simulink model "ms2"  (R2023b)
settings: Solver=FixedStepDiscrete  StartTime=0.0  StopTime=10.0  FixedStep=1e-3  RelTol=1e-3  EnableMultiTasking=on
settings Model: DataDictionary=common.sldd  Creator=mfussi  LastModifiedBy=mfussi
settings SolverCC: AutoInsertRateTranBlk=on  InsertRTBMode=Never (minimum delay)
settings DataIOCC: SaveOutput=off  SignalLogging=off  DSMLogging=off  StreamToWks=off  SaveTime=off  ReturnWorkspaceOutputs=off
settings OptimizationCC: DefaultParameterBehavior=Inlined  UseDivisionForNetSlopeComputation=on  GainParamInheritBuiltInType=on  UseFloatMulNetSlope=on  InlineInvariantSignals=on  EnhancedBackFolding=on  NoFixptDivByZeroProtection=on  EfficientFloat2IntCast=on  OptimizeBlockOrder=speed  DifferentSizesBufferReuse=on  OptimizationCustomize=off  EfficientTunableParamExpr=on
settings DebuggingCC: ParameterTunabilityLossMsg=error
settings HardwareCC: ProdBitPerPointer=32  ProdBitPerSizeT=32  ProdBitPerPtrDiffT=32  ProdLargestAtomicInteger=Long  ProdLargestAtomicFloat=Double  ProdWordSize=32  ProdLongLongMode=on  ProdHWDeviceType=ARM Compatible->ARM Cortex-M
settings SFSimCC: MATLABDynamicMemAlloc=off
settings SFSimCC: SimCustomHeaderCode=|
  | #include "rtw_enable_disable_motors.h"
  | #include "rtw_motor_config.h"
settings SFSimCC: SimUserSources=|
  | rtw_enable_disable_motors.c
  | rtw_motor_config.c
settings RTWCC: Description=Embedded Coder  SystemTargetFile=ert.tlc  GenCodeOnly=on  TemplateMakefile=ert_default_tmf  RTWUseSimCustomCode=on
settings RTWCC: CustomHeaderCode=|
  | #include "rtw_enable_disable_motors.h"
  | #include "rtw_motor_config.h"
settings RTWCC: CustomSource=|
  | rtw_enable_disable_motors.c
  | rtw_motor_config.c
settings CodeAppCC: ForceParamTrailComments=on  IgnoreCustomStorageClasses=off  OperatorAnnotations=on  SimulinkDataObjDesc=on  SFDataObjDesc=on  InsertBlockDesc=on
settings ERTTargetCC: TargetLangStandard=C99 (ISO)  CodeReplacementLibrary=ARM Cortex-M,iCubTech  GenerateSampleERTMain=on  SuppressErrorStatus=on  CodeInterfacePackaging=Reusable function  SupportNonFinite=off  InlinedParameterPlacement=NonHierarchical  RootIOFormat=Structure reference  ERTCustomFileTemplate=example_file_process.tlc

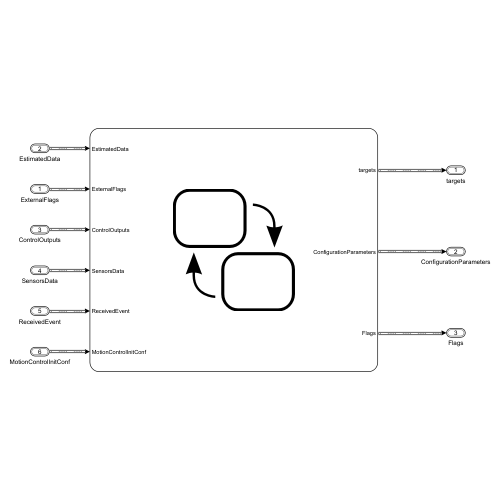
[thumbnail: Simulink's stored preview of the top-level diagram]
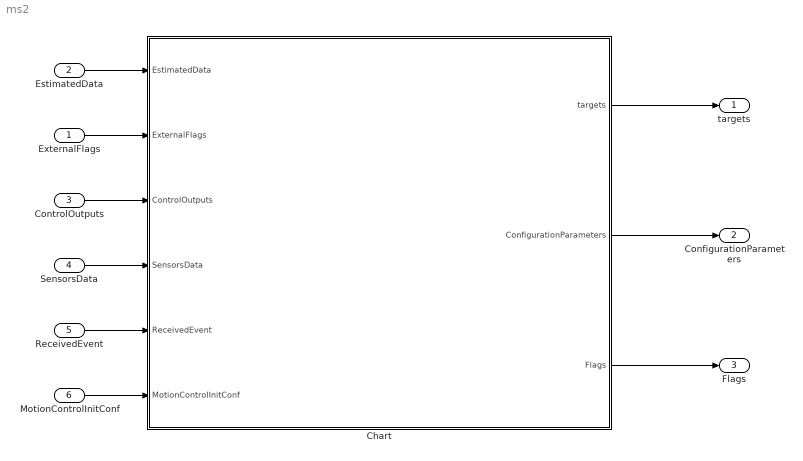
== system ms2 ==
  ExternalFlags : Inport  OutDataTypeStr=Bus: ExternalFlags  BusOutputAsStruct=on
  EstimatedData : Inport  Port=2  OutDataTypeStr=Bus: EstimatedData  BusOutputAsStruct=on
  ControlOutputs : Inport  Port=3  OutDataTypeStr=Bus: FOCOutputs  BusOutputAsStruct=on
  SensorsData : Inport  Port=4  OutDataTypeStr=Bus: SensorsData  BusOutputAsStruct=on
  ReceivedEvent : Inport  Port=5  OutDataTypeStr=Bus: SupervisorReceivedEvents  BusOutputAsStruct=on
  MotionControlInitConf : Inport  Port=6  OutDataTypeStr=Bus: ActuatorConfiguration  BusOutputAsStruct=on
  Chart : Stateflow chart  TreatAsAtomicUnit=on
  targets : Outport  OutDataTypeStr=Bus: Targets  BusOutputAsStruct=on
  ConfigurationParameters : Outport  Port=2  OutDataTypeStr=Bus: ActuatorConfiguration  BusOutputAsStruct=on
  Flags : Outport  Port=3  OutDataTypeStr=Bus: Flags  BusOutputAsStruct=on
  wires:
  ExternalFlags/1 -> Chart/2(ExternalFlags)
  EstimatedData/1 -> Chart/1(EstimatedData)
  ControlOutputs/1 -> Chart/3(ControlOutputs)
  SensorsData/1 -> Chart/4(SensorsData)
  ReceivedEvent/1 -> Chart/5(ReceivedEvent)
  Chart/1(targets) -> targets/1
  Chart/2(ConfigurationParameters) -> ConfigurationParameters/1
  Chart/3(Flags) -> Flags/1
  MotionControlInitConf/1 -> Chart/6(MotionControlInitConf)

== stateflow chart ms2/Chart ==
  settings: updateMethod=DISCRETE  sampleTime=1e-3
  state FaultsManager [parallel]
    settings: executionOrder=1
    state FaultButton [parallel]
      settings: executionOrder=2
      state NoFault
        entry:
        isFaultButtonPressed = false;
      state ButtonPressed
        entry:
        isFaultButtonPressed = true;
        send(faultButtonPressed, ControlModeHandler);
      (default) -> FaultsManager.FaultButton.NoFault
      ButtonPressed -> FaultsManager.FaultButton.NoFault : [hasChangedTo(ExternalFlags.fault_button, false)]
      FaultsManager.FaultButton.NoFault -> ButtonPressed : [hasChangedTo(ExternalFlags.fault_button, true)]
    state HWFaults [parallel]
      settings: executionOrder=1
      state NoFault
        entry:
        //MotorFaultFlags.overCurrent=0;
      state LimitNonConfigured
      state OverCurrentFault
        entry:
        //MotorFaultFlags.overCurrent=1;
        isInFault=true;
        send(hwFault, ControlModeHandler);
      (default) -> LimitNonConfigured
      LimitNonConfigured -> FaultsManager.HWFaults.NoFault : [areLimitsSet==true]
      FaultsManager.HWFaults.NoFault -> OverCurrentFault : [abs(EstimatedData.Iq_filtered) >= ConfigurationParameters.thresholds.motorOverloadCurrents]
      OverCurrentFault -> FaultsManager.HWFaults.NoFault : [abs(EstimatedData.Iq_filtered) < ConfigurationParameters.thresholds.motorOverloadCurrents]
  state ControlModeHandler [parallel]
    settings: executionOrder=3
    state NotConfigured
      entry:
      Flags.control_mode = ControlModes.NotConfigured;
      // rtw_disableMotor();
    state Idle
      entry:
      Flags.control_mode = ControlModes.Idle;
      // rtw_disableMotor();
      //rtw_enableMotor()
      //this updates the targets value
      send(ControlModeSetpointChange, TargetsManager);
    state Position
      entry:
      Flags.control_mode = ControlModes.Position;
      newSetpoint=SensorsData.jointpositions;
      send(ControlModeSetpointChange, TargetsManager);
    state Current
      entry:
      Flags.control_mode = ControlModes.Current;
      send(ControlModeSetpointChange, TargetsManager);
    state HWFault
      entry:
      Flags.control_mode = ControlModes.HwFaultCM;
      // rtw_disableMotor();
      //this updates the targets value
      send(ControlModeSetpointChange, TargetsManager);
    state Voltage
      entry:
      Flags.control_mode = ControlModes.Voltage;
      send(ControlModeSetpointChange, TargetsManager);
    note: IMPORTANT:
        | Currently we use IDLE command to exit from HWFault state,
        | but We should use FORCE_IDLE command when it will be implemented
    state Velocity
      entry:
      Flags.control_mode = ControlModes.Velocity;
      newSetpoint=0;
      send(ControlModeSetpointChange, TargetsManager);
    (junction 223) -> (junction 199)
    (junction 226) -> (junction 223) [order 1] : initialControlModeTrigger
    (junction 199) -> (junction 233)
    (default) -> (junction 226)
    (junction 226) -> NotConfigured [order 2]
    NotConfigured -> (junction 229) [order 1] : initialControlModeTrigger
        | {requiredControlMode = ControlModes.Idle;}
    (junction 229) -> (junction 233)
    (junction 227) -> (junction 233)
    (junction 282) -> (junction 227)
    (junction 273) -> (junction 229)
    (junction 233) -> Idle
    HWFault -> NotConfigured [order 1] : [!isInFault && isReqMode(ControlModes.Idle) && !isConfigurationSet()]
    NotConfigured -> HWFault [order 2] : [isInFault]
    (junction 228) -> Idle
    (junction 236) -> (junction 228)
    Idle -> (junction 230) [order 2]
    (junction 230) -> (junction 237)
    (junction 234) -> Idle : SetCtrlMode[isReqMode(ControlModes.Idle)]
    (junction 235) -> (junction 234) [order 2]
    (junction 224) -> Idle : SetCtrlMode[isReqMode(ControlModes.Idle)]
    (junction 243) -> (junction 224) [order 2]
    (junction 231) -> Idle : SetCtrlMode[isReqMode(ControlModes.Idle)]
    (junction 241) -> (junction 231) [order 2]
    Idle -> (junction 232) [order 1] : [isInFault || isFaultButtonPressed]
    (junction 232) -> (junction 225)
    (junction 225) -> (junction 248)
    Position -> (junction 236) [order 3] : SetCtrlMode[isReqMode(ControlModes.Idle)]
    (junction 237) -> Position [order 1] : SetCtrlMode[isReqMode(ControlModes.Position)]
    (junction 237) -> (junction 244) [order 2]
    (junction 235) -> Position [order 1] : SetCtrlMode[isReqMode(ControlModes.Position)]
    (junction 245) -> (junction 235)
    Position -> (junction 242) [order 2] : SetCtrlMode[!isReqMode(ControlModes.Idle)]
    (junction 242) -> (junction 240)
    (junction 243) -> Position [order 1] : SetCtrlMode[isReqMode(ControlModes.Position)]
    (junction 247) -> (junction 243) [order 2]
    (junction 241) -> Position [order 1] : SetCtrlMode[isReqMode(ControlModes.Position)]
    (junction 255) -> (junction 241) [order 2]
    Position -> (junction 238) [order 1] : [isInFault || isFaultButtonPressed]
    (junction 238) -> (junction 248)
    (junction 248) -> (junction 259)
    (junction 244) -> Current [order 1] : SetCtrlMode[isReqMode(ControlModes.Current)]{ newSetpoint=0; }
    (junction 244) -> (junction 278) [order 2]
    Current -> (junction 245) [order 3]
    (junction 240) -> (junction 239) [order 1] : SetCtrlMode[isReqMode(ControlModes.Current)]
    (junction 239) -> Current : {newSetpoint=ControlOutputs.Iq_fbk;}
    (junction 240) -> (junction 258) [order 2]
    (junction 247) -> (junction 246) [order 1] : SetCtrlMode[isReqMode(ControlModes.Current)]
    (junction 246) -> (junction 276)
    (junction 263) -> (junction 247)
    Current -> (junction 275) [order 2] : SetCtrlMode[!isReqMode(ControlModes.Idle) && !isReqMode(ControlModes.Position)]
    (junction 275) -> (junction 257)
    (junction 276) -> Current : {newSetpoint=ControlOutputs.Iq_fbk;}
    (junction 255) -> (junction 276) [order 1] : SetCtrlMode[isReqMode(ControlModes.Current)]
    HWFault -> (junction 273) [order 2] : SetCtrlMode[!isInFault && isReqMode(ControlModes.Idle)]
    (junction 261) -> (junction 255) [order 2]
    Current -> (junction 267) [order 1] : [isInFault || isFaultButtonPressed]
    (junction 267) -> (junction 259)
    (junction 259) -> (junction 279)
    (junction 268) -> HWFault
    (junction 278) -> Voltage [order 1] : SetCtrlMode[isReqMode(ControlModes.Voltage)]{newSetpoint=0; }
    (junction 278) -> (junction 251) [order 2]
    (junction 258) -> (junction 277) [order 1] : SetCtrlMode[isReqMode(ControlModes.Voltage)]
    (junction 277) -> Voltage : {newSetpoint=ControlOutputs.Vq;}
    (junction 258) -> (junction 251) [order 2]
    (junction 283) -> (junction 277)
    Voltage -> (junction 263) [order 2]
    (junction 257) -> (junction 283) [order 1] : SetCtrlMode[isReqMode(ControlModes.Voltage)]
    (junction 257) -> (junction 251) [order 2]
    Voltage -> (junction 251) [order 3]
    (junction 269) -> Voltage : {newSetpoint=ControlOutputs.Vq;}
    (junction 261) -> (junction 269) [order 1] : SetCtrlMode[isReqMode(ControlModes.Voltage)]
    (junction 265) -> (junction 261) : SetCtrlMode[!isReqMode(ControlModes.Velocity)]
    Voltage -> (junction 260) [order 1] : [isInFault || isFaultButtonPressed]
    (junction 260) -> (junction 279)
    (junction 279) -> (junction 253)
    (junction 251) -> Velocity : SetCtrlMode[isReqMode(ControlModes.Velocity)]
    Velocity -> (junction 265) [order 2]
    Velocity -> (junction 280) [order 1] : [isInFault || isFaultButtonPressed]
    (junction 280) -> (junction 253)
    (junction 253) -> (junction 281)
    (junction 281) -> (junction 268) [order 1] : [isInFault]
    (junction 281) -> (junction 282) [order 2] : [isFaultButtonPressed]
  state InputsDispatcher [parallel]
    settings: executionOrder=2
    state Target
      note: The idea here is : first of all reset all the targets and then set only the value of the given setpoint. If we are in idel or HW fault all targets remain equal to 0.
      (junction 814) -> (junction 812) [order 1] : [in(ControlModeHandler.Voltage)]{newSetpoint = ReceivedEvent.targets_content.motorvoltage;}
      (junction 812) -> (junction 813)
      (default) -> (junction 815)
      (junction 814) -> (junction 813) [order 2] : [in(ControlModeHandler.Current)]{newSetpoint = ReceivedEvent.targets_content.motorcurrent;}
      (junction 813) -> (junction 817)
      (junction 815) -> (junction 814) : [ReceivedEvent.event_type ==SupervisorEvents.SetTarget]
      (junction 814) -> (junction 817) [order 3] : [in(ControlModeHandler.Velocity)]{newSetpoint = ReceivedEvent.targets_content.jointvelocities;}
      (junction 814) -> (junction 818) [order 4] : {newSetpoint = 0;}
      (junction 817) -> (junction 818)
      (junction 818) -> (junction 819) : {send(DispatcherSetpointChange, TargetsManager);}
    state Waiting
    state Limits
      (default) -> (junction 788) : {ConfigurationParameters.thresholds=MotionControlInitConf.thresholds;}
      (junction 788) -> (junction 786) : [ReceivedEvent.limits_content.type == ControlModes.Current]
          | {ConfigurationParameters.thresholds.motorNominalCurrents = abs(ReceivedEvent.limits_content.nominal);
          | ConfigurationParameters.thresholds.motorPeakCurrents = abs(ReceivedEvent.limits_content.peak);
          | ConfigurationParameters.thresholds.motorOverloadCurrents = abs(ReceivedEvent.limits_content.overload);}
      (junction 786) -> (junction 784) : [areLimitsSet == false]
          | {areLimitsSet = true;
          | send(initialControlModeTrigger, ControlModeHandler);}
    state PID
      (default) -> (junction 874) : {ConfigurationParameters.pids.positionPID = MotionControlInitConf.pids.positionPID;}
      (junction 874) -> (junction 872) [order 5]
      (junction 874) -> (junction 878) [order 4] : [ReceivedEvent.pid_content.type == ControlModes.Velocity]
      (junction 874) -> (junction 877) [order 3] : [ReceivedEvent.pid_content.type == ControlModes.Voltage]
      (junction 874) -> (junction 875) [order 1] : [ReceivedEvent.pid_content.type == ControlModes.Current]
      (junction 872) -> (junction 879)
      (junction 874) -> (junction 876) [order 2] : [ReceivedEvent.pid_content.type == ControlModes.Position]
      (junction 876) -> (junction 884) : {ConfigurationParameters.pids.positionPID.P = 9;
          | ConfigurationParameters.pids.positionPID.I = 15;
          | ConfigurationParameters.pids.positionPID.D = 7;
          | ConfigurationParameters.pids.positionPID.shift_factor = ReceivedEvent.pid_content.shift_factor;
          | ConfigurationParameters.pids.positionPID.type = ControlModes.Position;}
      (junction 877) -> (junction 882) : {DirectPID.P = ReceivedEvent.pid_content.P;
          | DirectPID.I = ReceivedEvent.pid_content.I;
          | DirectPID.D = ReceivedEvent.pid_content.D;
          | DirectPID.shift_factor = ReceivedEvent.pid_content.shift_factor;}
      (junction 878) -> (junction 880) : {ConfigurationParameters.pids.velocityPID.P = ReceivedEvent.pid_content.P;
          | ConfigurationParameters.pids.velocityPID.I = ReceivedEvent.pid_content.I;
          | ConfigurationParameters.pids.velocityPID.D = ReceivedEvent.pid_content.D;
          | ConfigurationParameters.pids.velocityPID.shift_factor = ReceivedEvent.pid_content.shift_factor;}
      (junction 875) -> (junction 881) : {ConfigurationParameters.pids.currentPID.P = ReceivedEvent.pid_content.P;
          | ConfigurationParameters.pids.currentPID.I = ReceivedEvent.pid_content.I;
          | ConfigurationParameters.pids.currentPID.D = ReceivedEvent.pid_content.D;
          | ConfigurationParameters.pids.currentPID.shift_factor = ReceivedEvent.pid_content.shift_factor;
          | ConfigurationParameters.pids.currentPID.type = ControlModes.Current;}
      (junction 879) -> (junction 880)
      (junction 880) -> (junction 882)
      (junction 882) -> (junction 884)
      (junction 881) -> (junction 884)
    (default) -> Waiting
    Waiting -> Waiting [order 3] : [ReceivedEvent.event_type == SupervisorEvents.SetControlMode]
        | {send(SetCtrlMode, ControlModeHandler);
        | requiredControlMode=ReceivedEvent.control_mode_content;}
    Waiting -> Limits [order 1] : [ReceivedEvent.event_type == SupervisorEvents.SetLimit]
    Target -> Waiting
    Waiting -> Target [order 4] : [ReceivedEvent.event_type == SupervisorEvents.SetTarget]
    Limits -> Waiting
    PID -> Waiting
    Waiting -> PID [order 2] : [ReceivedEvent.event_type == SupervisorEvents.SetPid]
  state TargetsManager [parallel]
    settings: executionOrder=4
    state Home
    (default) -> Home : {targets.motorvoltage = 0;
        | targets.motorcurrent = 0;
        | targets.jointvelocities = 0;
        | targets.jointpositions = 0;}
    (junction 968) -> Home [order 1] : [in(ControlModeHandler.Current)]
        | {targets.motorcurrent = newSetpoint;}
    (junction 968) -> Home [order 4] : [in(ControlModeHandler.Position)]
        | {targets.jointpositions = newSetpoint;}
    (junction 968) -> Home [order 3] : [in(ControlModeHandler.Velocity)]
        | {targets.jointvelocities = newSetpoint;}
    (junction 968) -> Home [order 2] : [in(ControlModeHandler.Voltage)]
        | {targets.motorvoltage = newSetpoint;}
    Home -> (junction 968) [order 2] : DispatcherSetpointChange
    (junction 968) -> Home [order 5]
    Home -> (junction 968) [order 1] : ControlModeSetpointChange
  data: isSet function_output boolean; mode function_input double; out function_output double; areLimitsSet local boolean; EstimatedData input Bus: EstimatedData; ExternalFlags input Bus: ExternalFlags; ControlOutputs input Bus: FOCOutputs; targets output Bus: Targets; SensorsData input Bus: SensorsData; isFaultButtonPressed local double; ReceivedEvent input Bus: SupervisorReceivedEvents; isInFault local double; requiredControlMode local Enum: ControlModes; newSetpoint local double; DirectPID local Bus: PID; ConfigurationParameters output Bus: ActuatorConfiguration; Flags output Bus: Flags; MotionControlInitConf input Bus: ActuatorConfiguration
  events: initialControlModeTrigger local FUNCTION_CALL_EVENT; ControlModeSetpointChange local FUNCTION_CALL_EVENT; hwFault local FUNCTION_CALL_EVENT; faultButtonPressed local FUNCTION_CALL_EVENT; SetCtrlMode local FUNCTION_CALL_EVENT; DispatcherSetpointChange local FUNCTION_CALL_EVENT
  function isSet = isConfigurationSet:
    | function isSet = isConfigurationSet
    | 
    | % TODO: Add more conditions as more CAN packets are processed.
    | isSet = areLimitsSet; % && IsVoltageLimitSet && IsTemperatureLimitSet;
    | %isSet = isSet && a;
    | end
  function out=isReqMode(mode):
    | function out=isReqMode(mode)
    |    
    | if(requiredControlMode == mode)
    |     out=1;
    | else
    |     out=0;
    | end
